simulink model "ADP_1LinkRobot_PEFree_ModFree_Nash"  (Simulink 8.0)
settings: Solver=ode1  StartTime=0.0  StopTime=10  FixedStep=1/1000  RelTol=1e-3  AbsTol=1e-3
InitFcn:
  | ADP_1LinkRobot_PEFree_ModFree_Nash_PreSim
undefined symbols (not defined in the file): beta_1, beta_2, DY1, DY2, etaa1_1, etaa1_2, etaa2_1, etaa2_2, etac1_1, etac1_2, etac2_1, etac2_2, F, fs, g, Gamma0_1, Gamma0_2, GammaBar_1, GammaBar_2, GammaTheta, GG1, GG12, GG2, GG21, k, kTheta, L, learning, M, model, N, n, pecutoff, PHIPY, Q_1, Q_2, R_11, R_12, R_21, R_22, test, theta0, v_1, v_2, WaH0_1, WaH0_2, WcH0_1, WcH0_2, x0, XQX1, XQX2
settings Model: Creator=rkamalapurkar  LastModifiedBy=rkamalapurkar
settings DataIOCC: LimitDataPoints=off  MaxDataPoints=10000  SignalLoggingSaveFormat=ModelDataLogs
settings DebuggingCC: FcnCallInpInsideContextMsg=UseLocalSettings
settings CodeAppCC: CustomSymbolStrType=$N$R$M_T
settings GRTTargetCC: CombineOutputUpdateFcns=off  GRTInterface=on

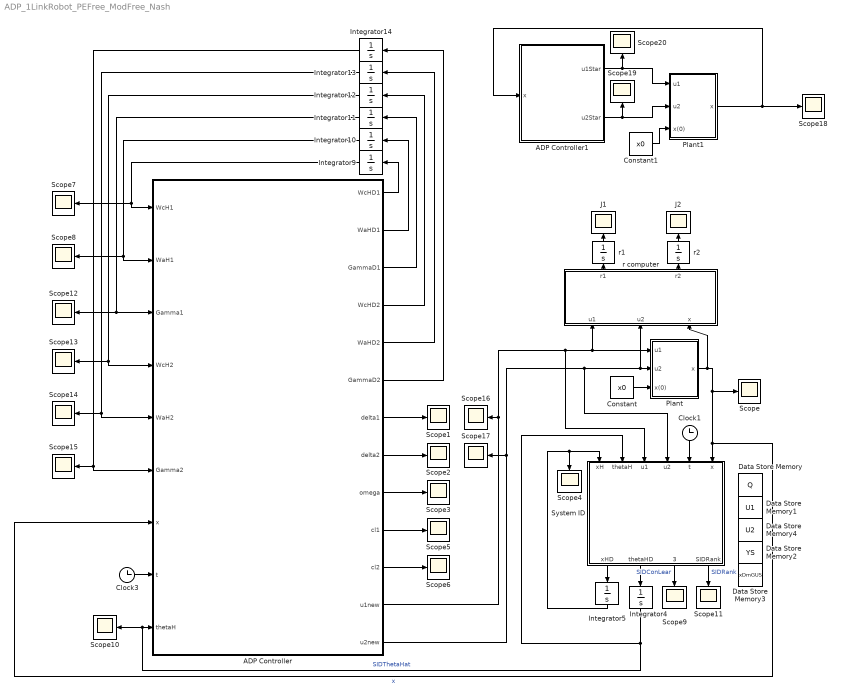
== system ADP_1LinkRobot_PEFree_ModFree_Nash ==
  ADP Controller : MATLAB Function  TreatAsAtomicUnit=on
      settings: PermitHierarchicalResolution=ParametersOnly
  ADP Controller1 : MATLAB Function  TreatAsAtomicUnit=on
      settings: PermitHierarchicalResolution=ParametersOnly
  Clock1 : Clock
  Clock3 : Clock
  Constant : Constant  Value=x0
  Constant1 : Constant  Value=x0
  Data Store Memory : DataStoreMemory  DataStoreName=Q  InitialValue=zeros(n,F)  OutDataTypeStr=double
  Data Store Memory1 : DataStoreMemory  DataStoreName=U1  InitialValue=zeros(1,(F+1)/2)  OutDataTypeStr=double
  Data Store Memory2 : DataStoreMemory  DataStoreName=YS  InitialValue=zeros(DY2,DY1*M)  OutDataTypeStr=double
  Data Store Memory3 : DataStoreMemory  DataStoreName=xDmGUS  InitialValue=zeros(n,M)  OutDataTypeStr=double
  Data Store Memory4 : DataStoreMemory  DataStoreName=U2  InitialValue=zeros(1,(F+1)/2)  OutDataTypeStr=double
  Integrator10 : Integrator  InitialCondition=WaH0_1
  Integrator11 : Integrator  InitialCondition=Gamma0_1
  Integrator12 : Integrator  InitialCondition=WcH0_2
  Integrator13 : Integrator  InitialCondition=WaH0_2
  Integrator14 : Integrator  InitialCondition=Gamma0_2
  Integrator4 : Integrator  InitialCondition=theta0
  Integrator5 : Integrator  InitialCondition=zeros(n,1)
  Integrator9 : Integrator  InitialCondition=WcH0_1
  J1 : Scope
      settings: YMin=2.75775e+007  YMax=2.76175e+007  SaveName=ScopeData14
  J2 : Scope
      settings: SaveName=ScopeData15
  Plant : Subsystem
  Plant1 : Subsystem
  Scope{,1..20} (21 alike) : Scope
      Scope settings: YMin=-12  YMax=1  SaveName=x
      Scope1 settings: YMin=-0.115  YMax=-0.03
      Scope10 settings: YMin=-2.25  YMax=1.25  SaveName=ThetaH
      Scope11 settings: YMin=0  YMax=1e-006  SaveName=cl1
      Scope12 settings: SaveName=ScopeData8
      Scope13 settings: YMin=-0.025  YMax=0.525  SaveName=WcH2
      Scope14 settings: YMin=-0.25  YMax=0.6  SaveName=WaH2
      Scope15 settings: TimeRange=0.5  YMin=-100  YMax=500  SaveName=ScopeData11
      Scope16 settings: YMin=-1.17  YMax=-0.98  SaveName=u1
      Scope17 settings: SaveName=u2
      Scope18 settings: YMin=-0.115  YMax=-0.03  SaveName=xStar
      Scope19 settings: YMin=-0.115  YMax=-0.03  SaveName=u2Star
      Scope20 settings: YMin=-0.115  YMax=-0.03  SaveName=u1Star
      Scope3 settings: SaveName=ScopeData2
      Scope4 settings: YMin=0  YMax=8.5e-05  SaveName=ScopeData3
      Scope5 settings: YMin=-3.5  YMax=0.75  SaveName=ScopeData4
      Scope6 settings: TimeRange=100  YMin=100  YMax=1000  SaveName=ScopeData5
      Scope7 settings: YMin=-1.25  YMax=1.75  SaveName=WcH1
      Scope8 settings: YMin=-0.05  YMax=1  SaveName=WaH1
      Scope9 settings: YMin=-1.6  YMax=0.4  SaveName=cl
  System ID : MATLAB Function  TreatAsAtomicUnit=on
      settings: PermitHierarchicalResolution=ParametersOnly
  r computer : MATLAB Function  TreatAsAtomicUnit=on
      settings: PermitHierarchicalResolution=ParametersOnly
  r1 : Integrator
  r2 : Integrator
  wires:
  Plant/1(x) -> System ID/6(x), ADP Controller/7(x), Scope/1, r computer/3(x)  "x"
  Constant/1 -> Plant/3(x(0))
  System ID/1(xHD) -> Integrator5/1
  System ID/4(SIDRank) -> Scope11/1  "SIDRank"
  System ID/3(SIDConLear) -> Scope9/1  "SIDConLear"
  System ID/2(thetaHD) -> Integrator4/1
  Clock1/1 -> System ID/5(t)
  Integrator5/1 -> System ID/1(xH), Scope4/1
  Integrator4/1 -> Scope10/1, ADP Controller/9(thetaH), System ID/2(thetaH)  "SIDThetaHat"
  ADP Controller/1(WcHD1) -> Integrator9/1
  ADP Controller/2(WaHD1) -> Integrator10/1
  ADP Controller/3(GammaD1) -> Integrator11/1
  ADP Controller/4(WcHD2) -> Integrator12/1
  ADP Controller/5(WaHD2) -> Integrator13/1
  ADP Controller/6(GammaD2) -> Integrator14/1
  ADP Controller/13(u2new) -> Scope17/1, System ID/4(u2), Plant/2(u2), r computer/2(u2)
  ADP Controller/12(u1new) -> Scope16/1, System ID/3(u1), Plant/1(u1), r computer/1(u1)
  Clock3/1 -> ADP Controller/8(t)
  ADP Controller/7(delta1) -> Scope1/1
  ADP Controller/8(delta2) -> Scope2/1
  ADP Controller/9(omega) -> Scope3/1
  ADP Controller/10(cl1) -> Scope5/1
  ADP Controller/11(cl2) -> Scope6/1
  Integrator9/1 -> ADP Controller/1(WcH1), Scope7/1
  Integrator10/1 -> ADP Controller/2(WaH1), Scope8/1
  Integrator11/1 -> Scope12/1, ADP Controller/3(Gamma1)
  Integrator12/1 -> ADP Controller/4(WcH2), Scope13/1
  Integrator13/1 -> ADP Controller/5(WaH2), Scope14/1
  Integrator14/1 -> ADP Controller/6(Gamma2), Scope15/1
  r computer/1(r1) -> r1/1
  r computer/2(r2) -> r2/1
  r1/1 -> J1/1
  r2/1 -> J2/1
  ADP Controller1/2(u2Star) -> Plant1/2(u2), Scope19/1
  ADP Controller1/1(u1Star) -> Scope20/1, Plant1/1(u1)
  Constant1/1 -> Plant1/3(x(0))
  Plant1/1(x) -> ADP Controller1/1(x), Scope18/1

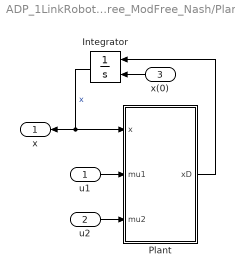
== system ADP_1LinkRobot_PEFree_ModFree_Nash/Plant ==
  u1 : Inport
  u2 : Inport  Port=2
  x(0) : Inport  Port=3
  Integrator : Integrator  InitialConditionSource=external  InitialCondition=[1;1;0.0;0.0]
  Plant : MATLAB Function  TreatAsAtomicUnit=on
      settings: PermitHierarchicalResolution=ParametersOnly
  x : Outport
  wires:
  Plant/1(xD) -> Integrator/1
  u1/1 -> Plant/2(mu1)
  x(0)/1 -> Integrator/2
  Integrator/1 -> Plant/1(x), x/1  "x"
  u2/1 -> Plant/3(mu2)

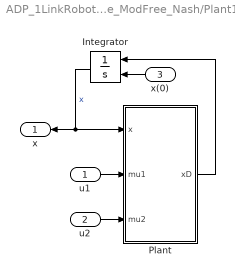
== system ADP_1LinkRobot_PEFree_ModFree_Nash/Plant1 ==
  u1 : Inport
  u2 : Inport  Port=2
  x(0) : Inport  Port=3
  Integrator : Integrator  InitialConditionSource=external  InitialCondition=[1;1;0.0;0.0]
  Plant : MATLAB Function  TreatAsAtomicUnit=on
      settings: PermitHierarchicalResolution=ParametersOnly
  x : Outport
  wires:
  Plant/1(xD) -> Integrator/1
  u1/1 -> Plant/2(mu1)
  x(0)/1 -> Integrator/2
  Integrator/1 -> Plant/1(x), x/1  "x"
  u2/1 -> Plant/3(mu2)

== matlab function Plant/Plant ==
  data: xD output double; x input double; mu1 input double; mu2 input double
function xD = dynamics(x,mu1,mu2)
%#codegen
F=[x(2)-2*x(1) ;-0.5*x(1)-x(2)+.25*x(2)*(cos(2*x(1))+2)^2+0.25*x(2)*(sin(4*x(1)^2)+2)^2];
G1=[0; cos(2*x(1))+2];
G2=[0; sin(4*x(1)^2)+2];
xD = F+G1*mu1+G2*mu2;

== matlab function r computer ==
  data: u1 input double; u2 input double; x input double; r1 output double; Q_1 parameter double; Q_2 parameter double; R_11 parameter double; R_21 parameter double; R_22 parameter double; R_12 parameter double; r2 output double
function [r1,r2] = getr(u1,u2,x,Q_1,Q_2,R_11,R_21,R_22,R_12)
%#codegen

r1 = x'*Q_1*x + u1'*R_11*u1 + u2'*R_21*u2;
r2 = x'*Q_2*x + u1'*R_12*u1 + u2'*R_22*u2;

end

== matlab function ADP Controller1 ==
  data: x input double; R_11 parameter double; R_22 parameter double; u1Star output double; u2Star output double
function [u1Star,u2Star]=OptimalControl(x,R_11,R_22)
%#codegen
W1 = [0.5;0;1];
W2 = [0.25;0;0.5];
G1 = [0 ; cos(2*x(1))+2];
G2 = [0 ; sin(4*x(1)^2)+2]; 
phi_p =[2*x(1) 0; x(2) x(1); 0 2*x(2)];
u1Star = -0.5*(R_11\G1')*phi_p'*W1;
u2Star = -0.5*(R_22\G2')*phi_p'*W2;

== matlab function System ID ==
  data: xH input double; xHD output double; thetaH input double; thetaHD output double; u1 input double; u2 input double; SIDConLear output double; SIDRank output double; t input double; x input double; k parameter double; GammaTheta parameter double; M parameter double; Q data_store_memory double; fs parameter double; F parameter double; g parameter double; YS data_store_memory double; xDmGUS data_store_memory double; U1 data_store_memory double; DY1 parameter double; kTheta parameter double; U2 data_store_memory double; model parameter double
function [xHD,thetaHD,SIDConLear,SIDRank] = SysID(xH,thetaH,u1,u2,t,x,k,...
    GammaTheta,M,fs,F,g,DY1,kTheta,model)
%#codegen
% This simulink block implements concurrent-learning based system
% identification using a Savitzky–Golay smoothing filter for state
% derivative computation. 
% fs: Sampling frequency
% M: number of stored data points
% F: Savitzky–Golay filter window length
% g: Savitzky–Golay filter differentiation matrix

global Q; % Data store memory for storing the values of x
global U1; % Data store memory for storing the values of u1
global U2; % Data store memory for storing the values of u2
global YS; % Data store memory for storing the values of Y,
           % made of Y' matrices stacked in a row
global xDmGUS; % Data store memory for storing the values of xDot - G*u

if model==0

n=round(t*fs)+1; % Current iteration number

xT = x-xH; % XTilde

%Dynamics
G1 = [0 ; cos(2*x(1))+2];
G2 = [0 ; sin(4*x(1)^2)+2]; 
Y = [x(2) x(1) 0 0 0 0 ;0 0 x(1) x(2) x(2)*(cos(2*x(1))+2)^2 x(2)*(sin(4*x(1)^2)+2)^2];

% For the first M points, store the values of Y and G*u
if n<=M
    YS(:,DY1*n-(DY1-1):DY1*n)=Y';
    xDmGUS(:,n)=G1*u1+G2*u2; % This will be subtracted from xDot later.
end

% At every time n store the past F values of the state. Note that 
% Q*g(:,2)/(1/fs) gives the state derivative at n-(F-1)/2
if n<=F
    Q(:,n)=x;
else
    Q = [Q(:,2:F) x];
end

% At every time n store the past (F+1)/2 values of the control. Actually, 
% we only need the value of u at n-(F-1)/2. However, I could not find a way
% to store just that single value. Also, even if U is initialized as a row
% vector, MATLAB seems to think its a column.
if n<=(F+1)/2
    U1(n)=u1;
    U2(n)=u2;
else
    U1 = [U1(2:(F+1)/2); u1];
    U2 = [U2(2:(F+1)/2); u2];
end

% Since the state derivative information is only available if n>=F and at 
% each time n, we can compute the state derivative evaluated at time 
% n-(F-1)/2, at time M+(F-1)/2, we we can evaluate the values of the state
% derivative at time steps from F-(F-1)/2 to M. Which in turn means that at
% this point we have M-(F+1)/2 usable values of XDot - G*u in the data
% store xDnGUs. The first (F-1)/2 values in xDmGUS are not usable.

index=0; 
nSt = (F+1)/2; % This is the starting index of usable values (=1+(F-1)/2)
if n<=M+(F-1)/2
    if n>=F % 
        xDj=Q*g(:,2)/(1/fs); % This is the state derivative at n-(F-1)/2
        xDmGUS(:,(n-(F-1)/2))=xDj-xDmGUS(:,(n-(F-1)/2));
    end
else 

% When n>M+(F-1)/2, use singular value maximization algorithm to replace
% elements of YS and XDmGUS with new data. At each time n, the value of the 
% state at n-(F-1)/2 can be found in Q(:,(F+1)/2)
    xj=Q(:,(F+1)/2); 
    Yj = [xj(2) xj(1) 0 0 0 0;0 0 xj(1) xj(2) xj(2)*(cos(2*xj(1))+2)^2 xj(2)*(sin(4*xj(1)^2)+2)^2];
    REGste1 = YS(:,DY1*nSt-(DY1-1):DY1*M)*YS(:,DY1*nSt-(DY1-1):DY1*M)';
    svd1=min(svd(REGste1)); % Minimum singular value of existing data
    for i=nSt:M
        te=YS; % Store existing data in a temporary variable
        te(:,DY1*i-(DY1-1):DY1*i)=Yj'; % Replace i'th Y' matrix with Yj'
        REGste2 = te(:,DY1*nSt-(DY1-1):DY1*M)*te(:,DY1*nSt-(DY1-1):DY1*M)';
        svd2=min(svd(REGste2)); % Minimum singular value after replacement
        if svd1<svd2   % If replacement results in a higher singular value,
            index=i;   % note the index of replacement and
            svd1=svd2; % keep searching for an even higher singular value.          
        end
    end
    
% At this point, index points to the matrix Y' in the stack YS which, when
% replaced with the new matrix Yj', results in the highest singular value.
% If index=0, the new data point is discarded. Otherwise, the stack YS, and
% correspondingly the stack xDmGUS is updated with the new data point. Note
% that since there is a delay of (F-1)/2 for derivative computation, the
% "new" data point we are talking about is the one that was recorded 
% (F-1)/2 steps ago.
    if index ~= 0
        YS(:,DY1*index-(DY1-1):DY1*index)=Yj';
        uj1=U1(1,1);
        uj2=U2(1,1);
        xDj=Q*g(:,2)/(1/fs);
        Gj1 = [0 ; cos(2*xj(1))+2];
        Gj2 = [0 ; sin(4*xj(1)^2)+2];
        xDmGUS(:,index)=xDj-Gj1*uj1-Gj2*uj2;
    end
end

xHD = Y*thetaH + G1*u1 + G2*u2 + k*xT;

% Find the index nEn of the last usable data point. This is only relevent 
% when n <= M+(F-1)/2. Otherwise, nEn = M.
nEn = nSt;
if n<=M+(F-1)/2 && n>=F
    nEn = n-(F-1)/2;
elseif n>M+(F-1)/2
    nEn=M; 
end
nEn = min(nEn,M);

% Final computation for the concurrent learning-based component of the
% adaptive update law. The concurrent learning component is zero for the
% first F timesteps.
REGs = YS(:,DY1*nSt-(DY1-1):DY1*nEn)*YS(:,DY1*nSt-(DY1-1):DY1*nEn)'*(n>=F);
SIDRank = min(svd(REGs)); % For plots
REG1s = YS(:,DY1*nSt-(DY1-1):DY1*nEn)*...
    reshape(xDmGUS(:,nSt:nEn),DY1*(nEn-nSt+1),1)*(n>=F);
SIDConLear = (REG1s-REGs*thetaH)/(nEn-nSt+1);
thetaHD = GammaTheta*Y'*xT + kTheta*GammaTheta*SIDConLear;
else 
thetaHD = zeros(6,1);
xHD=zeros(2,1);
SIDConLear=zeros(6,1);
SIDRank=zeros(1,1);
end%%%%%%%%%%%%%%%%%%%%%%%%%%%%%%%%%%%%%%%%%%%%%%%%%%%%%%%%

== matlab function ADP Controller ==
  data: WcH1 input double; WaH1 input double; Gamma1 input double; WcH2 input double; WaH2 input double; Gamma2 input double; x input double; t input double; thetaH input double; tf parameter double; R_11 parameter double; R_22 parameter double; R_21 parameter double; R_12 parameter double; Q_1 parameter double; Q_2 parameter double; etaa1_1 parameter double; etaa2_1 parameter double; etaa1_2 parameter double; etaa2_2 parameter double; etac1_1 parameter double; etac2_1 parameter double; etac1_2 parameter double; etac2_2 parameter double; v_1 parameter double; v_2 parameter double; XQX1 parameter double; XQX2 parameter double; GG1 parameter double; GG2 parameter double; GG12 parameter double; GG21 parameter double; PHIPY parameter double; N parameter double; pecutoff parameter double; learning parameter double; WcHD1 output double; WaHD1 output double; GammaD1 output double; WcHD2 output double; WaHD2 output double; GammaD2 output double; delta1 output double; model parameter double; L parameter double; beta_1 parameter double; GammaBar_1 parameter double; delta2 output double; omega output double; cl1 output double; cl2 output double; u1new output double; u2new output double; beta_2 parameter double; GammaBar_2 parameter double; test parameter double
function [WcHD1,WaHD1,GammaD1,WcHD2,WaHD2,GammaD2,delta1,delta2,omega,cl1,cl2,u1new,u2new]=...
    control(WcH1,WaH1,Gamma1,WcH2,WaH2,Gamma2,x,t,thetaH,tf,...
    R_11,R_22,R_21,R_12,Q_1,Q_2,...
    etaa1_1,etaa2_1,etaa1_2,etaa2_2,etac1_1,etac2_1,etac1_2,etac2_2,v_1,v_2,...
    XQX1,XQX2,GG1,GG2,GG12,GG21,PHIPY,N,pecutoff,learning,model,L,...
    beta_1,GammaBar_1,beta_2,GammaBar_2,test)
%#codegen
thetaS=[1 -2 -.5 -1 .25 .25]'; % True values of SysID Parameters
G1 = [0 ; cos(2*x(1))+2];
G2 = [0 ; sin(4*x(1)^2)+2]; 
Y = [x(2) x(1) 0 0 0 0 ;0 0 x(1) x(2) x(2)*(cos(2*x(1))+2)^2 x(2)*(sin(4*x(1)^2)+2)^2];
phi_p =[2*x(1) 0; x(2) x(1); 0 2*x(2)];
% F=[x(2)-2*x(1) ;-0.5*x(1)-x(2)+.25*x(2)*(cos(2*x(1))+2)^2+0.25*x(2)*(sin(4*x(1)^2)+2)^2];
u1=-0.5*(R_11\G1')*phi_p'*WaH1;
u2=-0.5*(R_22\G2')*phi_p'*WaH2;
% pe = sin(2*pi*t) + sin(exp(1)*t) + cos(5*t)^5;
% pe = (1.2-exp(.01*t))*(cos(0.2*t)^2+(sin(2*t)^2)*cos(0.1*t)+(sin(-1.2*t)^2)*cos(0.5*t)+sin(t)^5);
pe = sin(2*pi*t) + sin(exp(1)*t) + cos(5*t)^5;% + (1.2-exp(.01*t))*(cos(0.2*t)^2+(sin(2*t)^2)*cos(0.1*t)+(sin(-1.2*t)^2)*cos(0.5*t)+sin(t)^5);
u1new = u1 + pe*(t<=tf*pecutoff)*(learning==2);
u2new = u2 + pe*(t<=tf*pecutoff)*(learning==2);

theta = thetaS*(model==1) + thetaH*(model~=1);
%% Concurrent Learning
PHIPYtheta = reshape(PHIPY*theta,L,N);
GGWaH1 = reshape(GG1*WaH1,L,N);
GGWaH2 = reshape(GG2*WaH2,L,N);
GGWaH12 = reshape(GG12*WaH2,L,N);
GGWaH21 = reshape(GG21*WaH1,L,N);
Omegac = PHIPYtheta-(1/2)*GGWaH1-(1/2)*GGWaH2;
% player 1
deltac1 = (PHIPYtheta')*WcH1 + XQX1-(1/2)*(GGWaH1'*WcH1)+(1/4)*(GGWaH1'*WaH1)-(1/2)*(GGWaH2'*WcH1)+(1/4)*(GGWaH12'*WaH2);
normm1 = 1./(1.+v_1.*dot(Omegac.',Omegac.'*Gamma1.',2));
Omegac1 = Omegac*diag(normm1);
cl1 = -etac2_1*Gamma1*Omegac1*deltac1/N;
% player 2
deltac2 = (PHIPYtheta')*WcH2 + XQX2-(1/2)*(GGWaH2'*WcH2)+(1/4)*(GGWaH2'*WaH2)-(1/2)*(GGWaH1'*WcH2)+(1/4)*(GGWaH21'*WaH1);
normm2 = 1./(1.+v_2.*dot(Omegac.',Omegac.'*Gamma2.',2));
Omegac2 = Omegac*diag(normm2);
cl2 = -etac2_2*Gamma2*Omegac2*deltac2/N;

%% ADP
omega = phi_p*(Y*theta+G1*u1+G2*u2);
% omega = phi_p*(F+G1*u1+G2*u2);
% player 1
Gsigma1 = phi_p*G1*(R_11\G1')*phi_p'; %
Gsigma12 = phi_p*G2*(1/R_22)*R_12*(1/R_22)*G2'*phi_p'; %
Gsigma21 = phi_p*G1*(1/R_11)*R_21*(1/R_11)*G1'*phi_p';
r1 = x'*Q_1*x + u1'*R_11*u1 + u2'*R_12*u2; %
delta1 = WcH1'*omega + r1;
rho1 = (1+v_1*omega'*(Gamma1)*omega);
rho2 = (1+v_2*omega'*(Gamma2)*omega);
WcHD1 = (-etac1_1*Gamma1*omega*delta1/rho1+cl1)*(test==0);
GammaD1 = (beta_1*Gamma1-etac1_1*Gamma1*(omega*omega'/rho1^2)*Gamma1)*(norm(Gamma1)<=GammaBar_1)*(test==0);
WaHD1 = (etaa1_1*(WcH1-WaH1)-etaa2_1*WaH1+etac1_1*Gsigma1'*WaH1*omega'*WcH1/(4*rho1)...
    +etac2_1*GGWaH1*Omegac1'*WcH1/(4*N)+...
    +etac1_2*Gsigma21'*WaH1*omega'*WcH2/(4*rho2)+...
    +etac2_2*GGWaH21*Omegac2'*WcH2/(4*N))*(test==0);
% player 2
Gsigma2 = phi_p*G2*(R_22\G2')*phi_p'; %
r2 = x'*Q_2*x + u1'*R_21*u1 + u2'*R_22*u2; %
delta2 = WcH2'*omega + r2;
WcHD2 = (-etac1_2*Gamma2*omega*delta2/rho2+cl2)*(test==0);
GammaD2 = (beta_2*Gamma2-etac1_2*Gamma2*(omega*omega'/rho2^2)*Gamma2)*(norm(Gamma2)<=GammaBar_2)*(test==0);
WaHD2 = (etaa1_2*(WcH2-WaH2)-etaa2_2*WaH2+etac1_2*Gsigma2'*WaH2*omega'*WcH2/(4*rho2)...
    +etac2_2*GGWaH2*Omegac2'*WcH2/(4*N)+...
    +etac1_1*Gsigma12'*WaH2*omega'*WcH1/(4*rho2)+...
    +etac2_1*GGWaH12*Omegac1'*WcH1/(4*N))*(test==0);


end

== matlab function Plant1/Plant ==
  data: xD output double; x input double; mu1 input double; mu2 input double
function xD = dynamics(x,mu1,mu2)
%#codegen
F=[x(2)-2*x(1) ;-0.5*x(1)-x(2)+.25*x(2)*(cos(2*x(1))+2)^2+0.25*x(2)*(sin(4*x(1)^2)+2)^2];
G1=[0; cos(2*x(1))+2];
G2=[0; sin(4*x(1)^2)+2];
xD = F+G1*mu1+G2*mu2;
